simulink model "a1_stairs"  (R2022b)
settings: Solver=VariableStepAuto  StartTime=0.0  StopTime=5  FixedStep=0.001  MaxStep=Auto  MinStep=Auto  RelTol=1e-3
values from neighbouring files (symbols this model uses):
  Astate = [A1; A2; A3; A4; A5; A6]    [AME556_HW4_Cornwell.m]    (also in AME_556_Final_Project.m)
  calfd = -1.6    [AME556_HW3_Cornwell.m]    (also in AME_556_Final_Project.m)
  dt = params.dt    [AME556_HW4_Cornwell.m]    (also in AME_556_Final_Project.m = 0.03)
  gait_type = 1    [AME_556_Final_Project.m]
  H = H3    [AME556_HW1_Cornwell.m]    (also in AME556_HW4_Cornwell.m = blkdiag(H,Rmpc); AME_556_Final_Project.m = blkdiag(H,Rmpc))
  hipd = 0    [AME556_HW3_Cornwell.m]    (also in AME_556_Final_Project.m)
  kd = params.kd    [AME556_HW3_Cornwell.m]    (also in AME_556_Final_Project.m = 4)
  kp = params.kp    [AME556_HW3_Cornwell.m]    (also in AME_556_Final_Project.m = 25)
  m = params.m    [AME556_HW3_Cornwell.m]    (also in AME556_HW4_Cornwell.m = params.mass)
  N = size(x, 2)    [AME556_HW3_Cornwell.m]    (also in AME556_HW4_Cornwell.m; AME_556_Final_Project.m = 10)
  PD = 0    [AME_556_Final_Project.m]
  Q = diag([40 50 60 10 10 10 4 4 4 1 1 1 0])    [AME556_HW4_Cornwell.m]    (also in AME_556_Final_Project.m = diag([0 800 15000 49500 14000 5000 1900 700 700 900 700 200 )
  speed = 0.37    [AME_556_Final_Project.m]
  thighd = 0.95    [AME556_HW3_Cornwell.m]    (also in AME_556_Final_Project.m)
  Tstance = 0.15    [AME_556_Final_Project.m]
  X = quadprog(H,f,Astate,bstate,Aeq,beq)    [AME556_HW4_Cornwell.m]
  z0 = [x0(1)-1; x0(2)]    [AME556_HW5_Cornwell.m]    (also in AME_556_Final_Project.m = 0.2855)
  zd = 0.31    [AME_556_Final_Project.m]
undefined symbols (not defined in the file or in its folder): Y, Z
libraries: sm_lib x211, nesl_utility x96
(part 5 of 6)

== system a1_stairs/Robot dog/RR_thigh ==
  Inertia : sm_lib/Body Elements/Inertia  InertiaType=Custom  Mass=1.013  MassUnits=kg  CenterOfMass=[0, 0, 0]  CenterOfMassUnits=m  MomentsOfInertia=[0.005529065, 0.005139339, 0.001367788]  MomentsOfInertiaUnits=kg*m^2  ProductsOfInertia=[-2.2448e-05, 0.000343869, -4.825e-06]  ProductsOfInertiaUnits=kg*m^2  GraphicType=None  MarkerShape=Inertia  MarkerSize=20  GraphicVisPropType=SimpleVisualProperties  GraphicDiffuseColor=[0.5 0.5 0.5]  GraphicSpecularColor=[0.5 0.5 0.5 1.0]  GraphicAmbientColor=[0.15 0.15 0.15 1.0]  GraphicEmissiveColor=[0.0 0.0 0.0 1.0]  GraphicShininess=75  GraphicOpacity=1.0
  InertiaOriginTransform : sm_lib/Frames and Transforms/Rigid Transform  TranslationMethod=Cartesian  TranslationStandardOffset=0  TranslationLengthUnit=m  TranslationStandardAxis=+Z  TranslationCartesianOffset=[-0.003237, 0.022327, -0.027326]  TranslationROffset=0  TranslationROffsetUnits=m  TranslationZOffset=0  TranslationZOffsetUnits=m  TranslationThetaOffset=0  TranslationThetaOffsetUnits=deg  RotationMethod=RotationSequence  RotationAngleUnits=deg  RotationStandardAxis=+Z  RotationAngle=0.0  RotationArbitraryAxis=[0 0 1]  FollAlignAxisA=+X  BaseAlignAxisA=+Y  FollAlignAxisB=+Y  BaseAlignAxisB=+Z  RotationSequenceAxes=BaseAxes  RotationSequence=XYZ  RotationSequenceAngles=[0, 0, 0]  RotationSequenceAnglesUnits=rad  RotationMatrix=[1 0 0; 0 1 0; 0 0 1]  Quaternion=[1 0 0 0]
  RR_calf_joint_AxisTransform : sm_lib/Frames and Transforms/Rigid Transform  TranslationMethod=Cartesian  TranslationStandardOffset=0  TranslationLengthUnit=m  TranslationStandardAxis=+Z  TranslationCartesianOffset=[0, 0, 0]  TranslationROffset=0  TranslationROffsetUnits=m  TranslationZOffset=0  TranslationZOffsetUnits=m  TranslationThetaOffset=0  TranslationThetaOffsetUnits=deg  RotationMethod=ArbitraryAxis  RotationAngleUnits=rad  RotationStandardAxis=+Z  RotationAngle=1.570796326794897  RotationArbitraryAxis=[-1, 0, 0]  FollAlignAxisA=+X  BaseAlignAxisA=+Y  FollAlignAxisB=+Y  BaseAlignAxisB=+Z  RotationSequenceAxes=FollowerAxes  RotationSequence=XYX  RotationSequenceAngles=[0 0 0]  RotationSequenceAnglesUnits=deg  RotationMatrix=[1 0 0; 0 1 0; 0 0 1]  Quaternion=[1 0 0 0]
  RR_calf_joint_OriginTransform : sm_lib/Frames and Transforms/Rigid Transform  TranslationMethod=Cartesian  TranslationStandardOffset=0  TranslationLengthUnit=m  TranslationStandardAxis=+Z  TranslationCartesianOffset=[0, 0, -0.2]  TranslationROffset=0  TranslationROffsetUnits=m  TranslationZOffset=0  TranslationZOffsetUnits=m  TranslationThetaOffset=0  TranslationThetaOffsetUnits=deg  RotationMethod=RotationSequence  RotationAngleUnits=deg  RotationStandardAxis=+Z  RotationAngle=0.0  RotationArbitraryAxis=[0 0 1]  FollAlignAxisA=+X  BaseAlignAxisA=+Y  FollAlignAxisB=+Y  BaseAlignAxisB=+Z  RotationSequenceAxes=BaseAxes  RotationSequence=XYZ  RotationSequenceAngles=[0, 0, 0]  RotationSequenceAnglesUnits=rad  RotationMatrix=[1 0 0; 0 1 0; 0 0 1]  Quaternion=[1 0 0 0]
  RR_thigh_joint_AxisInvTransform : sm_lib/Frames and Transforms/Rigid Transform  TranslationMethod=Cartesian  TranslationStandardOffset=0  TranslationLengthUnit=m  TranslationStandardAxis=+Z  TranslationCartesianOffset=[0, 0, 0]  TranslationROffset=0  TranslationROffsetUnits=m  TranslationZOffset=0  TranslationZOffsetUnits=m  TranslationThetaOffset=0  TranslationThetaOffsetUnits=deg  RotationMethod=ArbitraryAxis  RotationAngleUnits=rad  RotationStandardAxis=+Z  RotationAngle=1.570796326794897  RotationArbitraryAxis=[-1, 0, 0]  FollAlignAxisA=+X  BaseAlignAxisA=+Y  FollAlignAxisB=+Y  BaseAlignAxisB=+Z  RotationSequenceAxes=FollowerAxes  RotationSequence=XYX  RotationSequenceAngles=[0 0 0]  RotationSequenceAnglesUnits=deg  RotationMatrix=[1 0 0; 0 1 0; 0 0 1]  Quaternion=[1 0 0 0]
  ReferenceFrame : sm_lib/Frames and Transforms/Reference Frame
  Visual : sm_lib/Body Elements/File Solid  ExtGeomFileName=a1_description/meshes/thigh_mirror.stl  UnitType=Custom  ExtGeomFileUnits=m  StepReaderType=HEX  ExportConvexHullGeometry=off  InertiaType=Custom  Mass=0  MassUnits=kg  CenterOfMass=[0, 0, 0]  CenterOfMassUnits=m  MomentsOfInertia=[0, 0, 0]  MomentsOfInertiaUnits=kg*m^2  ProductsOfInertia=[0, 0, 0]  ProductsOfInertiaUnits=kg*m^2  BasedOnType=DensityFromFile  Density=1000  DensityUnits=kg/m^3  DoExposeReferenceFrame=on  SerializedFrames=<Frames/>  GraphicType=FromGeometry  MarkerShape=Sphere  MarkerSize=10  GraphicVisPropType=SimpleVisualProperties  GraphicDiffuseColor=[0.8 0.8 1.0]  GraphicSpecularColor=[0.5 0.5 0.5 1.0]  GraphicAmbientColor=[0.15 0.15 0.15 1.0]  GraphicEmissiveColor=[0.0 0.0 0.0 1.0]  GraphicShininess=75  GraphicOpacity=1
  VisualOriginTransform : sm_lib/Frames and Transforms/Rigid Transform  TranslationMethod=Cartesian  TranslationStandardOffset=0  TranslationLengthUnit=m  TranslationStandardAxis=+Z  TranslationCartesianOffset=[0, 0, 0]  TranslationROffset=0  TranslationROffsetUnits=m  TranslationZOffset=0  TranslationZOffsetUnits=m  TranslationThetaOffset=0  TranslationThetaOffsetUnits=deg  RotationMethod=RotationSequence  RotationAngleUnits=deg  RotationStandardAxis=+Z  RotationAngle=0.0  RotationArbitraryAxis=[0 0 1]  FollAlignAxisA=+X  BaseAlignAxisA=+Y  FollAlignAxisB=+Y  BaseAlignAxisB=+Z  RotationSequenceAxes=BaseAxes  RotationSequence=XYZ  RotationSequenceAngles=[0, 0, 0]  RotationSequenceAnglesUnits=rad  RotationMatrix=[1 0 0; 0 1 0; 0 0 1]  Quaternion=[1 0 0 0]
  F : PMIOPort  Side=Left
  F1 : PMIOPort  Port=2  Side=Right
  connections:
  Inertia/RConn1 -- InertiaOriginTransform/RConn1
  RR_calf_joint_AxisTransform/RConn1 -- F1/RConn1
  RR_calf_joint_AxisTransform/LConn1 -- RR_calf_joint_OriginTransform/RConn1
  RR_thigh_joint_AxisInvTransform/RConn1 -- F/RConn1
  RR_calf_joint_OriginTransform/LConn1 -- InertiaOriginTransform/LConn1 -- ReferenceFrame/RConn1 -- VisualOriginTransform/LConn1 -- RR_thigh_joint_AxisInvTransform/LConn1
  Visual/RConn1 -- VisualOriginTransform/RConn1

== system a1_stairs/Robot dog/RR_thigh_shoulder ==
  ReferenceFrame : sm_lib/Frames and Transforms/Reference Frame
  F : PMIOPort  Side=Left
  connections:
  ReferenceFrame/RConn1 -- F/RConn1

== system a1_stairs/Robot dog/base ==
  ReferenceFrame : sm_lib/Frames and Transforms/Reference Frame
  Visual : sm_lib/Body Elements/Brick Solid  GraphicAmbientColor=[0.15 0.15 0.15 1.0]  BasedOnType=Density  BrickDimensions=[0.001, 0.001, 0.001]  BrickDimensionUnits=m  CenterOfMass=[0, 0, 0]  CenterOfMassUnits=m  GraphicDiffuseColor=[0.5, 0.5, 0.5]  Density=1000  DensityUnits=kg/m^3  DoExposeReferenceFrame=on  GraphicEmissiveColor=[0.0 0.0 0.0 1.0]  ExportEntireGeometry=off  SerializedFrames=<Frames/>  MarkerShape=Sphere  MarkerSize=10  GraphicType=FromGeometry  InertiaType=Custom  Mass=0  MassUnits=kg  MomentsOfInertia=[0, 0, 0]  MomentsOfInertiaUnits=kg*m^2  GraphicOpacity=1  ProductsOfInertia=[0, 0, 0]  ProductsOfInertiaUnits=kg*m^2  GraphicShininess=75  GraphicSpecularColor=[0.5 0.5 0.5 1.0]  GraphicVisPropType=SimpleVisualProperties
  VisualOriginTransform : sm_lib/Frames and Transforms/Rigid Transform  TranslationMethod=Cartesian  TranslationStandardOffset=0  TranslationLengthUnit=m  TranslationStandardAxis=+Z  TranslationCartesianOffset=[0, 0, 0]  TranslationROffset=0  TranslationROffsetUnits=m  TranslationZOffset=0  TranslationZOffsetUnits=m  TranslationThetaOffset=0  TranslationThetaOffsetUnits=deg  RotationMethod=RotationSequence  RotationAngleUnits=deg  RotationStandardAxis=+Z  RotationAngle=0.0  RotationArbitraryAxis=[0 0 1]  FollAlignAxisA=+X  BaseAlignAxisA=+Y  FollAlignAxisB=+Y  BaseAlignAxisB=+Z  RotationSequenceAxes=BaseAxes  RotationSequence=XYZ  RotationSequenceAngles=[0, 0, 0]  RotationSequenceAnglesUnits=rad  RotationMatrix=[1 0 0; 0 1 0; 0 0 1]  Quaternion=[1 0 0 0]
  floating_base_OriginTransform : sm_lib/Frames and Transforms/Rigid Transform  TranslationMethod=Cartesian  TranslationStandardOffset=0  TranslationLengthUnit=m  TranslationStandardAxis=+Z  TranslationCartesianOffset=[0, 0, z0]  TranslationROffset=0  TranslationROffsetUnits=m  TranslationZOffset=0  TranslationZOffsetUnits=m  TranslationThetaOffset=0  TranslationThetaOffsetUnits=deg  RotationMethod=RotationSequence  RotationAngleUnits=deg  RotationStandardAxis=+Z  RotationAngle=0.0  RotationArbitraryAxis=[0 0 1]  FollAlignAxisA=+X  BaseAlignAxisA=+Y  FollAlignAxisB=+Y  BaseAlignAxisB=+Z  RotationSequenceAxes=BaseAxes  RotationSequence=XYZ  RotationSequenceAngles=[0, 0, 0]  RotationSequenceAnglesUnits=rad  RotationMatrix=[1 0 0; 0 1 0; 0 0 1]  Quaternion=[1 0 0 0]
  F : PMIOPort  Side=Left
  F1 : PMIOPort  Port=2  Side=Right
  connections:
  VisualOriginTransform/LConn1 -- ReferenceFrame/RConn1 -- F/RConn1 -- floating_base_OriginTransform/LConn1
  Visual/RConn1 -- VisualOriginTransform/RConn1
  floating_base_OriginTransform/RConn1 -- F1/RConn1

== system a1_stairs/Robot dog/imu_link ==
  Inertia : sm_lib/Body Elements/Inertia  InertiaType=Custom  Mass=0.001  MassUnits=kg  CenterOfMass=[0, 0, 0]  CenterOfMassUnits=m  MomentsOfInertia=[0.0001, 0.0001, 0.0001]  MomentsOfInertiaUnits=kg*m^2  ProductsOfInertia=[0, 0, 0]  ProductsOfInertiaUnits=kg*m^2  GraphicType=None  MarkerShape=Inertia  MarkerSize=20  GraphicVisPropType=SimpleVisualProperties  GraphicDiffuseColor=[0.5 0.5 0.5]  GraphicSpecularColor=[0.5 0.5 0.5 1.0]  GraphicAmbientColor=[0.15 0.15 0.15 1.0]  GraphicEmissiveColor=[0.0 0.0 0.0 1.0]  GraphicShininess=75  GraphicOpacity=1.0
  InertiaOriginTransform : sm_lib/Frames and Transforms/Rigid Transform  TranslationMethod=Cartesian  TranslationStandardOffset=0  TranslationLengthUnit=m  TranslationStandardAxis=+Z  TranslationCartesianOffset=[0, 0, 0]  TranslationROffset=0  TranslationROffsetUnits=m  TranslationZOffset=0  TranslationZOffsetUnits=m  TranslationThetaOffset=0  TranslationThetaOffsetUnits=deg  RotationMethod=RotationSequence  RotationAngleUnits=deg  RotationStandardAxis=+Z  RotationAngle=0.0  RotationArbitraryAxis=[0 0 1]  FollAlignAxisA=+X  BaseAlignAxisA=+Y  FollAlignAxisB=+Y  BaseAlignAxisB=+Z  RotationSequenceAxes=BaseAxes  RotationSequence=XYZ  RotationSequenceAngles=[0, 0, 0]  RotationSequenceAnglesUnits=rad  RotationMatrix=[1 0 0; 0 1 0; 0 0 1]  Quaternion=[1 0 0 0]
  ReferenceFrame : sm_lib/Frames and Transforms/Reference Frame
  Visual : sm_lib/Body Elements/Brick Solid  GraphicAmbientColor=[0.15 0.15 0.15 1.0]  BasedOnType=Density  BrickDimensions=[0.001, 0.001, 0.001]  BrickDimensionUnits=m  CenterOfMass=[0, 0, 0]  CenterOfMassUnits=m  GraphicDiffuseColor=[0.8, 0, 0]  Density=1000  DensityUnits=kg/m^3  DoExposeReferenceFrame=on  GraphicEmissiveColor=[0.0 0.0 0.0 1.0]  ExportEntireGeometry=off  SerializedFrames=<Frames/>  MarkerShape=Sphere  MarkerSize=10  GraphicType=FromGeometry  InertiaType=Custom  Mass=0  MassUnits=kg  MomentsOfInertia=[0, 0, 0]  MomentsOfInertiaUnits=kg*m^2  GraphicOpacity=1  ProductsOfInertia=[0, 0, 0]  ProductsOfInertiaUnits=kg*m^2  GraphicShininess=75  GraphicSpecularColor=[0.5 0.5 0.5 1.0]  GraphicVisPropType=SimpleVisualProperties
  VisualOriginTransform : sm_lib/Frames and Transforms/Rigid Transform  TranslationMethod=Cartesian  TranslationStandardOffset=0  TranslationLengthUnit=m  TranslationStandardAxis=+Z  TranslationCartesianOffset=[0, 0, 0]  TranslationROffset=0  TranslationROffsetUnits=m  TranslationZOffset=0  TranslationZOffsetUnits=m  TranslationThetaOffset=0  TranslationThetaOffsetUnits=deg  RotationMethod=RotationSequence  RotationAngleUnits=deg  RotationStandardAxis=+Z  RotationAngle=0.0  RotationArbitraryAxis=[0 0 1]  FollAlignAxisA=+X  BaseAlignAxisA=+Y  FollAlignAxisB=+Y  BaseAlignAxisB=+Z  RotationSequenceAxes=BaseAxes  RotationSequence=XYZ  RotationSequenceAngles=[0, 0, 0]  RotationSequenceAnglesUnits=rad  RotationMatrix=[1 0 0; 0 1 0; 0 0 1]  Quaternion=[1 0 0 0]
  F : PMIOPort  Side=Left
  connections:
  Inertia/RConn1 -- InertiaOriginTransform/RConn1
  ReferenceFrame/RConn1 -- InertiaOriginTransform/LConn1 -- VisualOriginTransform/LConn1 -- F/RConn1
  Visual/RConn1 -- VisualOriginTransform/RConn1

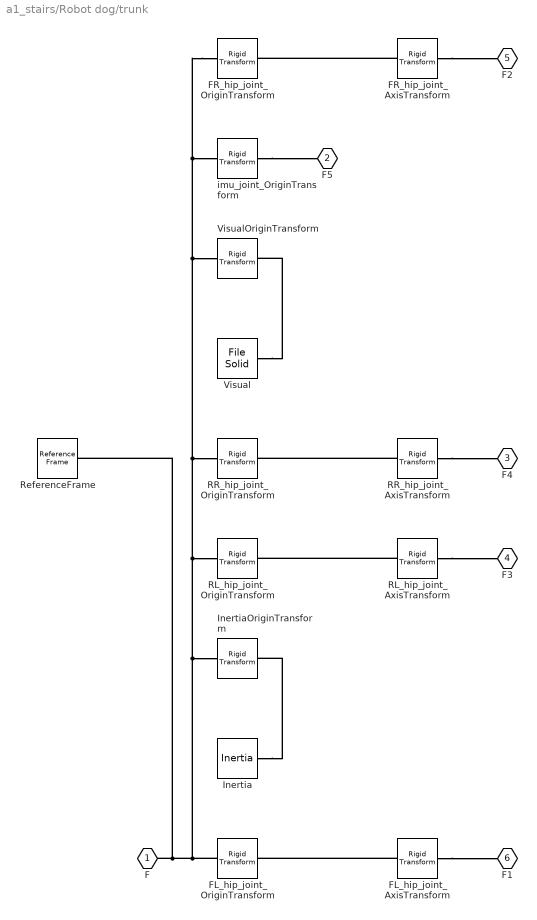
== system a1_stairs/Robot dog/trunk ==
  FL_hip_joint_AxisTransform : sm_lib/Frames and Transforms/Rigid Transform  TranslationMethod=Cartesian  TranslationStandardOffset=0  TranslationLengthUnit=m  TranslationStandardAxis=+Z  TranslationCartesianOffset=[0, 0, 0]  TranslationROffset=0  TranslationROffsetUnits=m  TranslationZOffset=0  TranslationZOffsetUnits=m  TranslationThetaOffset=0  TranslationThetaOffsetUnits=deg  RotationMethod=ArbitraryAxis  RotationAngleUnits=rad  RotationStandardAxis=+Z  RotationAngle=1.570796326794897  RotationArbitraryAxis=[-0, 1, 0]  FollAlignAxisA=+X  BaseAlignAxisA=+Y  FollAlignAxisB=+Y  BaseAlignAxisB=+Z  RotationSequenceAxes=FollowerAxes  RotationSequence=XYX  RotationSequenceAngles=[0 0 0]  RotationSequenceAnglesUnits=deg  RotationMatrix=[1 0 0; 0 1 0; 0 0 1]  Quaternion=[1 0 0 0]
  FL_hip_joint_OriginTransform : sm_lib/Frames and Transforms/Rigid Transform  TranslationMethod=Cartesian  TranslationStandardOffset=0  TranslationLengthUnit=m  TranslationStandardAxis=+Z  TranslationCartesianOffset=[0.1805, 0.047, 0]  TranslationROffset=0  TranslationROffsetUnits=m  TranslationZOffset=0  TranslationZOffsetUnits=m  TranslationThetaOffset=0  TranslationThetaOffsetUnits=deg  RotationMethod=RotationSequence  RotationAngleUnits=deg  RotationStandardAxis=+Z  RotationAngle=0.0  RotationArbitraryAxis=[0 0 1]  FollAlignAxisA=+X  BaseAlignAxisA=+Y  FollAlignAxisB=+Y  BaseAlignAxisB=+Z  RotationSequenceAxes=BaseAxes  RotationSequence=XYZ  RotationSequenceAngles=[0, 0, 0]  RotationSequenceAnglesUnits=rad  RotationMatrix=[1 0 0; 0 1 0; 0 0 1]  Quaternion=[1 0 0 0]
  FR_hip_joint_AxisTransform : sm_lib/Frames and Transforms/Rigid Transform  TranslationMethod=Cartesian  TranslationStandardOffset=0  TranslationLengthUnit=m  TranslationStandardAxis=+Z  TranslationCartesianOffset=[0, 0, 0]  TranslationROffset=0  TranslationROffsetUnits=m  TranslationZOffset=0  TranslationZOffsetUnits=m  TranslationThetaOffset=0  TranslationThetaOffsetUnits=deg  RotationMethod=ArbitraryAxis  RotationAngleUnits=rad  RotationStandardAxis=+Z  RotationAngle=1.570796326794897  RotationArbitraryAxis=[-0, 1, 0]  FollAlignAxisA=+X  BaseAlignAxisA=+Y  FollAlignAxisB=+Y  BaseAlignAxisB=+Z  RotationSequenceAxes=FollowerAxes  RotationSequence=XYX  RotationSequenceAngles=[0 0 0]  RotationSequenceAnglesUnits=deg  RotationMatrix=[1 0 0; 0 1 0; 0 0 1]  Quaternion=[1 0 0 0]
  FR_hip_joint_OriginTransform : sm_lib/Frames and Transforms/Rigid Transform  TranslationMethod=Cartesian  TranslationStandardOffset=0  TranslationLengthUnit=m  TranslationStandardAxis=+Z  TranslationCartesianOffset=[0.1805, -0.047, 0]  TranslationROffset=0  TranslationROffsetUnits=m  TranslationZOffset=0  TranslationZOffsetUnits=m  TranslationThetaOffset=0  TranslationThetaOffsetUnits=deg  RotationMethod=RotationSequence  RotationAngleUnits=deg  RotationStandardAxis=+Z  RotationAngle=0.0  RotationArbitraryAxis=[0 0 1]  FollAlignAxisA=+X  BaseAlignAxisA=+Y  FollAlignAxisB=+Y  BaseAlignAxisB=+Z  RotationSequenceAxes=BaseAxes  RotationSequence=XYZ  RotationSequenceAngles=[0, 0, 0]  RotationSequenceAnglesUnits=rad  RotationMatrix=[1 0 0; 0 1 0; 0 0 1]  Quaternion=[1 0 0 0]
  Inertia : sm_lib/Body Elements/Inertia  InertiaType=Custom  Mass=6  MassUnits=kg  CenterOfMass=[0, 0, 0]  CenterOfMassUnits=m  MomentsOfInertia=[0.0158533, 0.0377999, 0.0456542]  MomentsOfInertiaUnits=kg*m^2  ProductsOfInertia=[-2.75e-05, -6.109999999999999e-05, -3.66e-05]  ProductsOfInertiaUnits=kg*m^2  GraphicType=None  MarkerShape=Inertia  MarkerSize=20  GraphicVisPropType=SimpleVisualProperties  GraphicDiffuseColor=[0.5 0.5 0.5]  GraphicSpecularColor=[0.5 0.5 0.5 1.0]  GraphicAmbientColor=[0.15 0.15 0.15 1.0]  GraphicEmissiveColor=[0.0 0.0 0.0 1.0]  GraphicShininess=75  GraphicOpacity=1.0
  InertiaOriginTransform : sm_lib/Frames and Transforms/Rigid Transform  TranslationMethod=Cartesian  TranslationStandardOffset=0  TranslationLengthUnit=m  TranslationStandardAxis=+Z  TranslationCartesianOffset=[0, 0.0041, -0.0005]  TranslationROffset=0  TranslationROffsetUnits=m  TranslationZOffset=0  TranslationZOffsetUnits=m  TranslationThetaOffset=0  TranslationThetaOffsetUnits=deg  RotationMethod=RotationSequence  RotationAngleUnits=deg  RotationStandardAxis=+Z  RotationAngle=0.0  RotationArbitraryAxis=[0 0 1]  FollAlignAxisA=+X  BaseAlignAxisA=+Y  FollAlignAxisB=+Y  BaseAlignAxisB=+Z  RotationSequenceAxes=BaseAxes  RotationSequence=XYZ  RotationSequenceAngles=[0, 0, 0]  RotationSequenceAnglesUnits=rad  RotationMatrix=[1 0 0; 0 1 0; 0 0 1]  Quaternion=[1 0 0 0]
  RL_hip_joint_AxisTransform : sm_lib/Frames and Transforms/Rigid Transform  TranslationMethod=Cartesian  TranslationStandardOffset=0  TranslationLengthUnit=m  TranslationStandardAxis=+Z  TranslationCartesianOffset=[0, 0, 0]  TranslationROffset=0  TranslationROffsetUnits=m  TranslationZOffset=0  TranslationZOffsetUnits=m  TranslationThetaOffset=0  TranslationThetaOffsetUnits=deg  RotationMethod=ArbitraryAxis  RotationAngleUnits=rad  RotationStandardAxis=+Z  RotationAngle=1.570796326794897  RotationArbitraryAxis=[-0, 1, 0]  FollAlignAxisA=+X  BaseAlignAxisA=+Y  FollAlignAxisB=+Y  BaseAlignAxisB=+Z  RotationSequenceAxes=FollowerAxes  RotationSequence=XYX  RotationSequenceAngles=[0 0 0]  RotationSequenceAnglesUnits=deg  RotationMatrix=[1 0 0; 0 1 0; 0 0 1]  Quaternion=[1 0 0 0]
  RL_hip_joint_OriginTransform : sm_lib/Frames and Transforms/Rigid Transform  TranslationMethod=Cartesian  TranslationStandardOffset=0  TranslationLengthUnit=m  TranslationStandardAxis=+Z  TranslationCartesianOffset=[-0.1805, 0.047, 0]  TranslationROffset=0  TranslationROffsetUnits=m  TranslationZOffset=0  TranslationZOffsetUnits=m  TranslationThetaOffset=0  TranslationThetaOffsetUnits=deg  RotationMethod=RotationSequence  RotationAngleUnits=deg  RotationStandardAxis=+Z  RotationAngle=0.0  RotationArbitraryAxis=[0 0 1]  FollAlignAxisA=+X  BaseAlignAxisA=+Y  FollAlignAxisB=+Y  BaseAlignAxisB=+Z  RotationSequenceAxes=BaseAxes  RotationSequence=XYZ  RotationSequenceAngles=[0, 0, 0]  RotationSequenceAnglesUnits=rad  RotationMatrix=[1 0 0; 0 1 0; 0 0 1]  Quaternion=[1 0 0 0]
  RR_hip_joint_AxisTransform : sm_lib/Frames and Transforms/Rigid Transform  TranslationMethod=Cartesian  TranslationStandardOffset=0  TranslationLengthUnit=m  TranslationStandardAxis=+Z  TranslationCartesianOffset=[0, 0, 0]  TranslationROffset=0  TranslationROffsetUnits=m  TranslationZOffset=0  TranslationZOffsetUnits=m  TranslationThetaOffset=0  TranslationThetaOffsetUnits=deg  RotationMethod=ArbitraryAxis  RotationAngleUnits=rad  RotationStandardAxis=+Z  RotationAngle=1.570796326794897  RotationArbitraryAxis=[-0, 1, 0]  FollAlignAxisA=+X  BaseAlignAxisA=+Y  FollAlignAxisB=+Y  BaseAlignAxisB=+Z  RotationSequenceAxes=FollowerAxes  RotationSequence=XYX  RotationSequenceAngles=[0 0 0]  RotationSequenceAnglesUnits=deg  RotationMatrix=[1 0 0; 0 1 0; 0 0 1]  Quaternion=[1 0 0 0]
  RR_hip_joint_OriginTransform : sm_lib/Frames and Transforms/Rigid Transform  TranslationMethod=Cartesian  TranslationStandardOffset=0  TranslationLengthUnit=m  TranslationStandardAxis=+Z  TranslationCartesianOffset=[-0.1805, -0.047, 0]  TranslationROffset=0  TranslationROffsetUnits=m  TranslationZOffset=0  TranslationZOffsetUnits=m  TranslationThetaOffset=0  TranslationThetaOffsetUnits=deg  RotationMethod=RotationSequence  RotationAngleUnits=deg  RotationStandardAxis=+Z  RotationAngle=0.0  RotationArbitraryAxis=[0 0 1]  FollAlignAxisA=+X  BaseAlignAxisA=+Y  FollAlignAxisB=+Y  BaseAlignAxisB=+Z  RotationSequenceAxes=BaseAxes  RotationSequence=XYZ  RotationSequenceAngles=[0, 0, 0]  RotationSequenceAnglesUnits=rad  RotationMatrix=[1 0 0; 0 1 0; 0 0 1]  Quaternion=[1 0 0 0]
  ReferenceFrame : sm_lib/Frames and Transforms/Reference Frame
  Visual : sm_lib/Body Elements/File Solid  ExtGeomFileName=a1_description/meshes/trunk.stl  UnitType=Custom  ExtGeomFileUnits=m  StepReaderType=HEX  ExportConvexHullGeometry=off  InertiaType=Custom  Mass=0  MassUnits=kg  CenterOfMass=[0, 0, 0]  CenterOfMassUnits=m  MomentsOfInertia=[0, 0, 0]  MomentsOfInertiaUnits=kg*m^2  ProductsOfInertia=[0, 0, 0]  ProductsOfInertiaUnits=kg*m^2  BasedOnType=DensityFromFile  Density=1000  DensityUnits=kg/m^3  DoExposeReferenceFrame=on  SerializedFrames=<Frames/>  GraphicType=FromGeometry  MarkerShape=Sphere  MarkerSize=10  GraphicVisPropType=SimpleVisualProperties  GraphicDiffuseColor=[1.0 0.8 1.0]  GraphicSpecularColor=[0.5 0.5 0.5 1.0]  GraphicAmbientColor=[0.15 0.15 0.15 1.0]  GraphicEmissiveColor=[0.0 0.0 0.0 1.0]  GraphicShininess=75  GraphicOpacity=1
  VisualOriginTransform : sm_lib/Frames and Transforms/Rigid Transform  TranslationMethod=Cartesian  TranslationStandardOffset=0  TranslationLengthUnit=m  TranslationStandardAxis=+Z  TranslationCartesianOffset=[0, 0, 0]  TranslationROffset=0  TranslationROffsetUnits=m  TranslationZOffset=0  TranslationZOffsetUnits=m  TranslationThetaOffset=0  TranslationThetaOffsetUnits=deg  RotationMethod=RotationSequence  RotationAngleUnits=deg  RotationStandardAxis=+Z  RotationAngle=0.0  RotationArbitraryAxis=[0 0 1]  FollAlignAxisA=+X  BaseAlignAxisA=+Y  FollAlignAxisB=+Y  BaseAlignAxisB=+Z  RotationSequenceAxes=BaseAxes  RotationSequence=XYZ  RotationSequenceAngles=[0, 0, 0]  RotationSequenceAnglesUnits=rad  RotationMatrix=[1 0 0; 0 1 0; 0 0 1]  Quaternion=[1 0 0 0]
  imu_joint_OriginTransform : sm_lib/Frames and Transforms/Rigid Transform  TranslationMethod=Cartesian  TranslationStandardOffset=0  TranslationLengthUnit=m  TranslationStandardAxis=+Z  TranslationCartesianOffset=[0, 0, 0]  TranslationROffset=0  TranslationROffsetUnits=m  TranslationZOffset=0  TranslationZOffsetUnits=m  TranslationThetaOffset=0  TranslationThetaOffsetUnits=deg  RotationMethod=RotationSequence  RotationAngleUnits=deg  RotationStandardAxis=+Z  RotationAngle=0.0  RotationArbitraryAxis=[0 0 1]  FollAlignAxisA=+X  BaseAlignAxisA=+Y  FollAlignAxisB=+Y  BaseAlignAxisB=+Z  RotationSequenceAxes=BaseAxes  RotationSequence=XYZ  RotationSequenceAngles=[0, 0, 0]  RotationSequenceAnglesUnits=rad  RotationMatrix=[1 0 0; 0 1 0; 0 0 1]  Quaternion=[1 0 0 0]
  F : PMIOPort  Side=Left
  F5 : PMIOPort  Port=2  Side=Right
  F4 : PMIOPort  Port=3  Side=Right
  F3 : PMIOPort  Port=4  Side=Right
  F2 : PMIOPort  Port=5  Side=Right
  F1 : PMIOPort  Port=6  Side=Right
  connections:
  FL_hip_joint_AxisTransform/RConn1 -- F1/RConn1
  FL_hip_joint_AxisTransform/LConn1 -- FL_hip_joint_OriginTransform/RConn1
  FR_hip_joint_AxisTransform/RConn1 -- F2/RConn1
  FR_hip_joint_AxisTransform/LConn1 -- FR_hip_joint_OriginTransform/RConn1
  Inertia/RConn1 -- InertiaOriginTransform/RConn1
  RL_hip_joint_AxisTransform/RConn1 -- F3/RConn1
  RL_hip_joint_AxisTransform/LConn1 -- RL_hip_joint_OriginTransform/RConn1
  RR_hip_joint_AxisTransform/RConn1 -- F4/RConn1
  RR_hip_joint_AxisTransform/LConn1 -- RR_hip_joint_OriginTransform/RConn1
  FR_hip_joint_OriginTransform/LConn1 -- FL_hip_joint_OriginTransform/LConn1 -- ReferenceFrame/RConn1 -- F/RConn1 -- InertiaOriginTransform/LConn1 -- RL_hip_joint_OriginTransform/LConn1 -- RR_hip_joint_OriginTransform/LConn1 -- VisualOriginTransform/LConn1 -- imu_joint_OriginTransform/LConn1
  Visual/RConn1 -- VisualOriginTransform/RConn1
  imu_joint_OriginTransform/RConn1 -- F5/RConn1

== matlab function a1_stairs/MPC and QP/QP  ==
  settings: updateMethod=DISCRETE  sampleTime=0.001
  data: x input; pf input; Xd input; gait_type input; u output
% QP gait controller
function u = QP(x,pf,Xd,gait_type)
    if gait_type ~= 0 % not standing
        u = zeros(12,1);
    else
        % Foot positions
        pf_FL = [pf(1); pf(2); pf(3)];
        pf_FR = [pf(4); pf(5); pf(6)];
        pf_RL = [pf(7); pf(8); pf(9)];
        pf_RR = [pf(10); pf(11); pf(12)];
    
        % Robot parameters
        mass = 12;
        I = diag([0.0168, 0.0565, 0.064]);
        mu = 0.5;

        % Constants
        g = [0; 0; -9.81];
        kp_p = diag([10,10,1000]);
        kd_p = diag([200,200,200]);
        kp_o = diag([750,750,750]);
        kd_o = diag([500,500,500]);
        alpha = 0.001;
        S = diag([2,2,100,100,100,100]);

        % Get desired from Xd
        pd = [Xd(1); Xd(2); Xd(3)];
        Rd = eul2rotm([Xd(6),Xd(5),Xd(4)]);
        dpd = [Xd(7); Xd(8); Xd(9)];
        wd = [Xd(10); Xd(11); Xd(12)];
    
        % Rearrange to get x
        px = x(1); py = x(2); pz = x(3);
        p = [px;py;pz];

        roll = x(4); pitch = x(5); yaw = x(6);
        R = eul2rotm([yaw,pitch,roll]);

        dx = x(7); dy = x(8); dz = x(9);
        dp = [dx;dy;dz];
        
        wx = x(10); wy = x(11); wz = x(12);
        w = [wx;wy;wz];

        % PD controller
        ddp = kp_p*(pd-p) + kd_p*(dpd-dp);
        e = rotmat2vec3d(Rd*transpose(R));
        dwd = kp_o*e' + kd_o*(wd-w);

        % r vectors in world frame
        r1 = pf_FL - p; % ri = pf-p
        r2 = pf_FR - p;
        r3 = pf_RL - p;
        r4 = pf_RR - p;
    
        bd = [mass.*ddp+mass.*g; I*dwd];
        A = [eye(3) eye(3) eye(3) eye(3);
            0 -r1(3) r1(2) 0 -r2(3) r2(2) 0 -r3(3) r3(2) 0 -r4(3) r4(2);
            r1(3) 0 -r1(1) r2(3) 0 -r2(1) r3(3) 0 -r3(1) r4(3) 0 -r4(1);
            -r1(2) r1(1) 0 -r2(2) r2(1) 0 -r3(2) r3(1) 0 -r4(2) r4(1) 0];
    
        H = transpose(A)*S*A+alpha;
        f = transpose(-transpose(bd)*S*A);

        % Inequality constraints
        A1_Fz = [0 0 1];
        A1 = blkdiag(A1_Fz,A1_Fz,A1_Fz,A1_Fz);
        A2 = -A1;
        A3_Fx = [1 0 -mu];
        A3 = blkdiag(A3_Fx,A3_Fx,A3_Fx,A3_Fx);
        A4_Fx = [-1 0 -mu];
        A4 = blkdiag(A4_Fx,A4_Fx,A4_Fx,A4_Fx);
        A5_Fx = [0 1 -mu];
        A5 = blkdiag(A5_Fx,A5_Fx,A5_Fx,A5_Fx);
        A6_Fx = [0 -1 -mu];
        A6 = blkdiag(A6_Fx,A6_Fx,A6_Fx,A6_Fx);
        Aqp = [A1; A2; A3; A4; A5; A6];
        bqp = [500*ones(4,1); -10*ones(4,1); zeros(16,1)];
        
        % Solve
        options = optimoptions('quadprog','Display','off','Algorithm','active-set'); 
        x0 = zeros(length(H),1);
        u = zeros(12,1);
        u = quadprog(H,f,Aqp,bqp,[],[],[],[],x0,options);
    
    end

end

== matlab function a1_stairs/Gait table ==
  settings: sampleTime=dt
  data: t input; gait_table output; dt input; gait_type input
function gait_table = gait(t,dt,gait_type)
    N=10;
        
    if gait_type < 1 % standing
        gait_table = ones(4*N,1);
    else
        time = floor(t/dt)*dt;

        % Initialize
        gait_table = zeros(N*4,1);
    
        if gait_type < 7 || time < 6 % no flight phase

            if mod(time/dt,N) == 0                      % divisible by N (or =0)
                contact1 = [ones(1,N/2) zeros(1,N/2)];   % start at stance
                contact2 = [zeros(1,N/2) ones(1,N/2)];  % start at swing
            elseif mod(time/dt,N) == N/2
                contact1 = [zeros(1,N/2) ones(1,N/2)];
                contact2 = [ones(1,N/2) zeros(1,N/2)];
            elseif mod(time/dt,N) < N/2
                offset = floor(mod(time/dt,N));
                contact1 = [ones(1,N/2-offset) zeros(1,N/2) ones(1,offset)];
                contact2 = [zeros(1,N/2-offset) ones(1,N/2) zeros(1,offset)];
            elseif mod(time/dt,N) > N/2
                offset = abs(N/2 - floor(mod(time/dt,N)));
                contact1 = [zeros(1,N/2-offset) ones(1,N/2) zeros(1,offset)];
                contact2 = [ones(1,N/2-offset) zeros(1,N/2) ones(1,offset)];
            else
                error('problem with time')
                contact1 = [ones(1,N/2) zeros(1,N/2)];   % start at stance
                contact2 = [zeros(1,N/2) ones(1,N/2)];  % start at swing
            end

        else % 7 = running
            swing = 6;
            stance = 4;

            % CONTACT 1
            if mod(time/dt,N) == 0                          % divisible by N (or =0)
                contact1 = [ones(1,stance) zeros(1,swing)];  % start at stance
            elseif mod(time/dt,N) == stance % end of stance - switch to swing first
                contact1 = [zeros(1,swing) ones(1,stance)];
            elseif mod(time/dt,N) < stance % still stance
                offset = floor(mod(time/dt,N));
                contact1 = [ones(1,stance-offset) zeros(1,swing) ones(1,offset)];
            elseif mod(time/dt,N) > stance % in swing
                offset = abs(N/2 - floor(mod(time/dt,N)));
                contact1 = [zeros(1,swing-offset) ones(1,stance) zeros(1,offset)];
            else
                error('problem with time')
                contact1 = [ones(1,N/2) zeros(1,N/2)];   % start at stance
            end

            % CONTACT 2
            if mod(time/dt,N) == 0                          % divisible by N (or =0)
                contact2 = [zeros(1,swing) ones(1,stance)];  % start at swing
            elseif mod(time/dt,N) == swing % end of swing - switch to stance first
                contact2 = [ones(1,stance) zeros(1,swing)];
            elseif mod(time/dt,N) < swing % still swing
                offset = floor(mod(time/dt,N));
                contact2 = [zeros(1,swing-offset) ones(1,stance) zeros(1,offset)];
            elseif mod(time/dt,N) > swing % in stance
                offset = abs(N/2 - floor(mod(time/dt,N)));
                contact2 = [ones(1,stance-offset) zeros(1,swing) ones(1,offset)];
            else
                error('problem with time')
                contact2 = [zeros(1,N/2) ones(1,N/2)];  % start at swing
            end

        end

        for ii = 0:N-1
            for jj = [1 4] % legs
                gait_table(4*ii+jj,1) = contact1(ii+1);
            end
            for jj = [2 3]
                gait_table(4*ii+jj,1) = contact2(ii+1);
            end
        end
    end

end

== matlab function a1_stairs/Get desired/MATLAB Function3 ==
  settings: updateMethod=DISCRETE  sampleTime=0.001
  data: x input; Xd output; gait_type input; zd input; speed input; pf input; gait_table input; Xd_prev input
% gait_type values:
% 0 = stand still
% 1 = moving forward
% 2 = moving backward
% 3 = moving left
% 4 = moving right
% 5 = rotate to the lift
% 6 = rotate to the right

function Xd = get_desired_state(x, gait_type, zd, speed, pf, gait_table, Xd_prev)

    % calculate new state
    if gait_type < 1 % standing still
        Xd = [0; 0; zd;
              0; 0; 0;
              0; 0; 0;
              0; 0; 0;
              -9.81];
    elseif gait_type == 1 % moving forward
        current_s = Xd_prev(7);
        if x(1) < 1.2
            if current_s < speed % ramp up
                new_s = current_s + speed*0.0008;
            else
                new_s = speed;
            end
        else
            new_s = current_s + 0.0001;
        end

        % Change pitch angle wrt to estimated surface plane of stairs
        px = [pf(1); pf(4); pf(7); pf(10)];
        py = [pf(2); pf(5); pf(8); pf(11)];
        pz = [pf(3); pf(6); pf(9); pf(12)];
%         W = [ones(4,1), px, py];
%         a = pinv(transpose(W)*W)*transpose(W)*pz;
%         normal_v = [a(2); a(3); -1];
%         ang = atan2(norm(cross(normal_v,[0;0;-1])),dot(normal_v,[0;0;-1]));
        
        % Find the two stance legs
        if gait_table(1) == 1
            front = [pf(1);pf(2);pf(3)];
        else
            front = [pf(4);pf(5);pf(6)];
        end
        if gait_table(3) == 1
            rear = [pf(7);pf(8);pf(9)];
        else
            rear = [pf(10);pf(11);pf(12)];
        end
        ang = -atan((front(3)-rear(3))/(front(1)-rear(1)));

        % Update desired z position

        R = eul2rotm([x(6), x(5), x(4)]);
        pf_b = transpose(R)*[0;0;min(pz(1:2))];
        p_w = R*(pf_b+[0;0;zd]);
        z = p_w(3);

        Xd = [0; 0; z;
              0; ang; 0;
              new_s; 0; 0;
              0; 0; 0;
              -9.81];
    else
        error('missing Xd based on movement_state')
    end

end

== matlab function a1_stairs/FP controller/MATLAB Function7 ==
  settings: sampleTime=0.03
  data: t input; foot_pos_forces output; swing_front output; gait_type input; x input; zd_com input; p_foot input; v_foot input; p_hip input; Tstance input; movement_speed input; gait_table input; path1_prev input; path2_prev input; path3_prev input; path4_prev input; path1 output; path2 output; swing_front_prev input; path3 output; path4 output
function [foot_pos_forces, swing_front, path1, path2, path3, path4] = footpos(t, gait_type, x,...
    zd_com, p_foot, v_foot, p_hip, Tstance, movement_speed, gait_table, ...
    path1_prev, path2_prev, path3_prev, path4_prev, swing_front_prev)
    % t (1x1) is the current time
    % gait_type is a constant setting the current objective
        % 0 = stand still
        % 1 = moving forward
        % 2 = moving backward
        % 3 = moving left
        % 4 = moving right
        % 5 = rotate to the left
        % 6 = rotate to the right
    % p_com is the current position
    % v_com (3x1) is the current velocity
    % w_com (3x1) are the current angular velocities (yaw,pitch,roll)
    % zd_com (1x1) is the desired COM height
    % p_hip (8x1) are the x,y positions of each hip
    % p_foot (12x1) are the x,y,z positions of each foot
    % v_foot (12x1) are the velcoities of each foot in x,y,z
    % Tstance (1x1) is the total time of the stance phase
    % gait_table is (4x1) with  rows for each leg where 1=stance, 0=swing
    % paths are (3x100) matrices describing the desired foot trajectories of the swing feet

    p_com = [x(1);x(2);x(3)];   % position
    o_com = [x(4);x(5);x(6)];   % orientation
    v_com = [x(7);x(8);x(9)];   % velocity
    w_com = [x(10);x(11);x(12)];% ang. velocity

    len = 151; %len = Tstance*1000+1;

    FL = gait_table(1,1); % if 0, this leg is in swing (must be controlled here)
    FR = gait_table(2);
    RL = gait_table(3);
    RR = gait_table(4);
    num_swing = 4-(FL+FR+RL+RR);
 
    t_current = mod(t,Tstance); % tells us how far into the stance we are
    g = 9.81;
    h1 = 0.07;
    h2 = 0.13; % get over stair 1
    h3 = 0.235;
    h4 = 0.33;
    h5 = 0.425;
    h6 = 0.53; 
    
    if x(1) < 0.62 % before stairs
        z_max_F = h1; % maximum height that the foot reaches
        z_max_R = h1;
    elseif x(1) < 0.85 % approaching stair 2
        z_max_F = h2;
        z_max_R = h1;
    elseif x(1) < 1.05 % approaching stair 3
        z_max_F = h3;
        z_max_R = h1;
    elseif x(1) < 1.2 % approaching  stair 4
        z_max_F = h4;
        z_max_R = h2;
    elseif x(1) < 1.3
        z_max_R = h2;
        z_max_F = h5;
    elseif x(1) < 1.41 % approaching stair 5
        z_max_F = h5;
        z_max_R = h3;
    elseif x(1) < 1.55
        z_max_F = h6;
        z_max_R = h5;
    else
        z_max_F = h6;
        z_max_R = h6;
    end

%         k_turn = 0.1;
    kd = 12; % just z?

    if size(v_com,1) == 1
        v_com = v_com';
    end

    timestamp = [0,Tstance/2,Tstance];          % the 3 times that correspond to the initial foot position, the maximum height, and the final position
    tt = linspace(timestamp(1),timestamp(end),len); % get evenly spaced points to interpolate
    [~,closestIndex] = min(abs(tt-t_current));  % find the point that corresponds to this current time in the stance

    if gait_type < 1                       % standing
        foot_pos_forces = zeros(12,1);
        path1 = zeros(3,len);
        path2 = zeros(3,len);
        path3 = zeros(3,len);
        path4 = zeros(3,len);
        swing_front = 0;
    else
        vd_com = [movement_speed; 0; 0];
        k_step = 0.22;

        p_hip1 = [p_hip(1); p_hip(2); 0];    % FL  - hip projected onto ground
        p_foot1 = [p_foot(1); p_foot(2); p_foot(3)];
        v_foot1 = [v_foot(1); v_foot(2); v_foot(3)];
        p_hip2 = [p_hip(3); p_hip(4); 0];    % FR - hip projected onto ground
        p_foot2 = [p_foot(4); p_foot(5); p_foot(6)];
        v_foot2 = [v_foot(4); v_foot(5); v_foot(6)];
        p_hip3 = [p_hip(5); p_hip(6); 0];    % RL
        p_foot3 = [p_foot(7); p_foot(8); p_foot(9)];
        v_foot3 = [v_foot(7); v_foot(8); v_foot(9)];
        p_hip4 = [p_hip(7); p_hip(8); 0];    % RR
        p_foot4 = [p_foot(10); p_foot(11); p_foot(12)];
        v_foot4 = [v_foot(10); v_foot(11); v_foot(12)];


        if FL == 0                  % FL, RR are in swing
            swing_front = 1;
     
            kp1 = diag([200;260;200]);
            kp2 = diag([200;750;200]);

        else                        % FR, RL are in swing
            swing_front = 2;

            kp1 = diag([200;500;200]); % x, y, z (front leg)
            kp2 = diag([200;1800;200]); % (rear leg)
        end

        if swing_front == 1 % FL and RR are in swing
            if swing_front_prev == 1
                % not a new phase
                path1 = path1_prev;
                path4 = path4_prev;
            else
                pd_foot1 = p_hip1 + Tstance/2*v_com + k_step*(v_com-vd_com);
                pd_foot1(3,1) = p_foot1(3);
                pd_foot4 = p_hip4 + Tstance/2*v_com + k_step*(v_com-vd_com);
                pd_foot4(3,1) = p_foot4(3);

                path1_pre = getpath(p_foot1, pd_foot1, tt, z_max_F, timestamp);
                path4_pre = getpath(p_foot4, pd_foot4, tt, z_max_R, timestamp);

                % Check for collisions
                path1 = check_collision(path1_pre, p_foot1, pd_foot1, tt, timestamp, 1);
                path4 = check_collision(path4_pre, p_foot4, pd_foot4, tt, timestamp, 4);
            end
            path2 = path2_prev;
            path3 = path3_prev;
        elseif swing_front == 2
            if swing_front_prev == 2
                % not a new phase
                path2 = path2_prev;
                path3 = path3_prev;
            else
                pd_foot2 = p_hip2 + Tstance/2*v_com + k_step*(v_com-vd_com);
                pd_foot2(3,1) = p_foot2(3);
                pd_foot3 = p_hip3 + Tstance/2*v_com + k_step*(v_com-vd_com);
                pd_foot3(3,1) = p_foot3(3);

                path2_pre = getpath(p_foot2, pd_foot2, tt, z_max_F, timestamp);
                path3_pre = getpath(p_foot3, pd_foot3, tt, z_max_R, timestamp);

                % Check for collisions
                path2 = check_collision(path2_pre, p_foot2, pd_foot2, tt, timestamp, 2);
                path3 = check_collision(path3_pre, p_foot3, pd_foot3, tt, timestamp, 3);
            end
            path1 = path1_prev;
            path4 = path4_prev;
        else
            error('no swing')
            path1 = path1_prev;
            path2 = path2_prev;
            path3 = path3_prev;
            path4 = path4_prev;
        end

        % Calculate velocities based on desired position path
        velocities1 = zeros(3,len);
        velocities2 = zeros(3,len);
        velocities3 = zeros(3,len);
        velocities4 = zeros(3,len);
        for ii = 1:3
            velocities1(ii,:) = [0 diff(path1(ii,:))./diff(tt)];
            velocities2(ii,:) = [0 diff(path2(ii,:))./diff(tt)];
            velocities3(ii,:) = [0 diff(path3(ii,:))./diff(tt)];
            velocities4(ii,:) = [0 diff(path4(ii,:))./diff(tt)];
        end

        % F = kp *(pfd(current) - pf) + kd *(vd(current) - vf)
        force1 = kp1*(path1(:,closestIndex)-p_foot1)+kd*(velocities1(:,closestIndex)-v_foot1); % P for x,y,z; D for z only
        force2 = kp1*(path2(:,closestIndex)-p_foot2)+kd*(velocities2(:,closestIndex)-v_foot2);
        force3 = kp2*(path3(:,closestIndex)-p_foot3)+kd*(velocities3(:,closestIndex)-v_foot3);
        force4 = kp2*(path4(:,closestIndex)-p_foot4)+kd*(velocities4(:,closestIndex)-v_foot4);

        if FL == 0
            foot_pos_forces = [force1; zeros(6,1); force4]; % force should be 12x1
        else
            foot_pos_forces = [zeros(3,1); force2; force3; zeros(3,1)];
        end
       
    end

end

function path = getpath(p_foot, pd_foot, tt, z_max, timestamp)
        x = [p_foot(1), p_foot(1)+(pd_foot(1)-p_foot(1))/2, pd_foot(1)];
        y = [p_foot(2), p_foot(2)+(pd_foot(2)-p_foot(2))/2, pd_foot(2)];
        z = [p_foot(3), z_max, pd_foot(3)];
        xx = interp1(timestamp,x,tt,'spline');
        yy = interp1(timestamp,y,tt,'spline');
        zz = interp1(timestamp,z,tt,'spline');
        path = [xx;yy;zz];

end

function new_path = check_collision(path, p_foot, pd_foot, tt, timestamp, foot)
    stair1 = [0.85;0;0.1];
    stair2 = [stair1(1)+0.2;0;0.2];
    stair3 = [stair2(1)+0.2;0;0.3];
    stair4 = [stair3(1)+0.2;0;0.4];
    stair5 = [stair4(1)+0.2;0;0.5];

    if path(3,1) < 0.09
        current_stair = 0;
    elseif path(3,1) < 0.19
        current_stair = 1;
    elseif path(3,1) < 0.29
        current_stair = 2;
    elseif path(3,1) < 0.39
        current_stair = 3;
    elseif path(3,1) < 0.49
        current_stair = 4;
    else
        current_stair = 5;
    end
        
    if current_stair == 0
        if path(1,end) < stair1(1) - 0.05
            new_path = path;
        else % close so get new path to clear the step
            pd_foot(1) = stair1(1)+0.07;
            pd_foot(3) = stair1(3);
            new_path = getpath(p_foot, pd_foot, tt, stair1(3)+0.02, timestamp);
        end
    elseif current_stair == 1
        if path(1,end) < path(1,1) % prevent going backwards
            pd_foot = p_foot;
            new_path = getpath(p_foot, pd_foot, tt, stair1(3)+0.05, timestamp);
        elseif path(1,end) < stair2(1) - 0.05
            new_path = path;
        else % close so get new path to clear the step
            pd_foot(1) = stair2(1)+0.07;
            pd_foot(3) = stair2(3);
            new_path = getpath(p_foot, pd_foot, tt, stair2(3)+0.03, timestamp);
        end
    elseif current_stair == 2
        if foot == 3
            pd_foot(1) = stair3(1)+0.05;
            pd_foot(3) = stair3(3);
            new_path = getpath(p_foot, pd_foot, tt, stair3(3)+0.02, timestamp);
        elseif path(1,end) < path(1,1) % prevent going backwards
            pd_foot = p_foot;
            new_path = getpath(p_foot, pd_foot, tt, stair2(3)+0.05, timestamp);
        elseif path(1,end) < stair3(1) - 0.05
            new_path = path;
        else % close so get new path to clear the step
            pd_foot(1) = stair3(1)+0.07;
            pd_foot(3) = stair3(3);
            new_path = getpath(p_foot, pd_foot, tt, stair3(3)+0.02, timestamp);
        end
    elseif current_stair == 3
        if foot == 3
            pd_foot(1) = stair4(1)+0.05;
            pd_foot(3) = stair4(3);
            new_path = getpath(p_foot, pd_foot, tt, stair4(3)+0.07, timestamp);
        elseif path(1,end) < path(1,1) % prevent going backwards
            pd_foot = p_foot;
            new_path = getpath(p_foot, pd_foot, tt, stair3(3)+0.05, timestamp);
        elseif path(1,end) < stair4(1) - 0.05
            new_path = path;
        else % close so get new path to clear the step
            if foot == 1
                pd_foot(1) = stair4(1)+0.13;
            else
                pd_foot(1) = stair4(1)+0.09;
            end
            pd_foot(3) = stair4(3);
            new_path = getpath(p_foot, pd_foot, tt, stair4(3)+0.02, timestamp);
        end
    elseif current_stair == 4
        if foot == 2
            pd_foot(1) = stair5(1)+0.05;
            pd_foot(3) = stair5(3);
            new_path = getpath(p_foot, pd_foot, tt, stair5(3)+0.02, timestamp);
        elseif path(1,end) < path(1,1) % prevent going backwards
            pd_foot = p_foot;
            new_path = getpath(p_foot, pd_foot, tt, stair4(3)+0.05, timestamp);
        elseif path(1,end) < stair5(1) - 0.05
            new_path = path;
        else % close so get new path to clear the step
            pd_foot(1) = stair5(1)+0.07;
            pd_foot(3) = stair5(3);
            new_path = getpath(p_foot, pd_foot, tt, stair5(3)+0.02, timestamp);
        end
    else
        new_path = path;
    end
end

== matlab function a1_stairs/Robot dog/MATLAB Function ==
  data: Q input; eul output
function eul = fcn(Q)
    Q = Q';

    angles = quat2eul(Q);                   % yaw pitch roll
    eul = [angles(3); angles(2); angles(1)]; % roll pitch yaw

end

== matlab function a1_stairs/Robot dog/MATLAB Function5 ==
  data: R input; thetax output; thetay output; thetaz output
function [thetax,thetay,thetaz] = fcn(R)
    theta_zyx = rotm2eul(R);
    thetax = theta_zyx(3);
    thetay = theta_zyx(2);
    thetaz = theta_zyx(1);
end

== matlab function a1_stairs/Convert to torque ==
  settings: sampleTime=0.001
  data: J_FL input; J_FR input; J_RL input; J_RR input; gait_type input; tau input; PD input; x input; u_MPC input; u_FP input; u_QP input; t_FL output; t_FR output; t_RL output; t_RR output; gait_table input
function [t_FL, t_FR, t_RL, t_RR] = fcn(J_FL, J_FR, J_RL, J_RR, gait_type,...
    tau, PD, x, u_MPC, u_FP, u_QP, gait_table)

    % Rotation matrix from x
    R = eul2rotm([x(6),x(5),x(4)]);

    % Tau from PD controller


    % Initialize
    F1 = zeros(3,1);
    F2 = zeros(3,1);
    F3 = zeros(3,1);
    F4 = zeros(3,1);
    
    % Check if each foot is in stance (MPC) or swing (FP)
    if gait_type == 0
        if PD == 0
            F1(1:3,1) = u_QP(1:3);
            t_FL = -transpose(J_FL)*transpose(R)*F1;    % 1
        else
            t_FL = [tau(1);tau(2);tau(3)];
        end
    elseif gait_table(1,1) == 1 
        F1(1:3,1) = u_MPC(1:3);
        t_FL = -transpose(J_FL)*transpose(R)*F1;    % 1
    else
        F1(1:3,1) = u_FP(1:3);
        t_FL = transpose(J_FL)*transpose(R)*F1;    % 1
    end

    if gait_type == 0
        if PD == 0
            F2(1:3,1) = u_QP(4:6);
            t_FR = -transpose(J_FR)*transpose(R)*F2;    % 2
        else
            t_FR = [tau(4);tau(5);tau(6)];
        end
    elseif gait_table(2,1) == 1
        F2(1:3,1) = u_MPC(4:6);
        t_FR = -transpose(J_FR)*transpose(R)*F2;    % 2
    else
        F2(1:3,1) = u_FP(4:6);
        t_FR = transpose(J_FR)*transpose(R)*F2;    % 2
    end
    
    if gait_type == 0
        if PD == 0
            F3(1:3,1) = u_QP(7:9);
            t_RL = -transpose(J_RL)*transpose(R)*F3;    % 3
        else
            t_RL = [tau(7);tau(8);tau(9)];
        end
    elseif gait_table(3,1) == 1
        F3(1:3,1) = u_MPC(7:9);
        t_RL = -transpose(J_RL)*transpose(R)*F3;    % 3
    else
        F3(1:3,1) = u_FP(7:9);
        t_RL = transpose(J_RL)*transpose(R)*F3;    % 3
    end

    if gait_type == 0
        if PD == 0
            F4(1:3,1) = u_QP(10:12);
            t_RR = -transpose(J_RR)*transpose(R)*F4;    % 4
        else
            t_RR = [tau(10);tau(11);tau(12)];
        end
    elseif gait_table(4,1) == 1
        F4(1:3,1) = u_MPC(10:12);
        t_RR = -transpose(J_RR)*transpose(R)*F4;    % 4
    else
        F4(1:3,1) = u_FP(10:12);
        t_RR = transpose(J_RR)*transpose(R)*F4;    % 4
    end

end
